simulink model "OpenLoop_simulation"  (R2022b)
settings: Solver=VariableStepAuto  StartTime=0.0  StopTime=5  RelTol=1e-3
values from neighbouring files (symbols this model uses):
  b = 0    [step_response_nominal.m]
  L = 0.23e-3    (= 0.00023)    [step_response_nominal.m]
  R = 3.85    [step_response_nominal.m]
  Stepsize = 0.5    [step_response_nominal.m]    (also in step_response_our.m)
  Tcomp = 0.0005*Ts*14    (= 7e-06)    [step_response_nominal.m]    (also in step_response_our.m)
  Ts = 0.001    [step_response_nominal.m]    (also in step_response_our.m)
settings Model: Creator=Alex Zhen  LastModifiedBy=lenovo
settings SolverCC: ZeroCrossAlgorithm=Adaptive
settings DebuggingCC: IgnoredZcDiagnostic=none

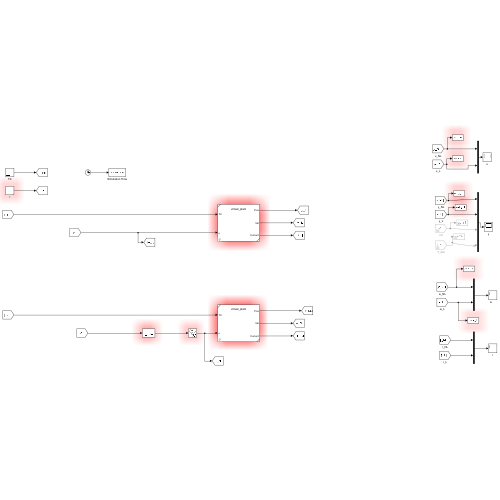
[thumbnail: Simulink's stored preview of the top-level diagram]
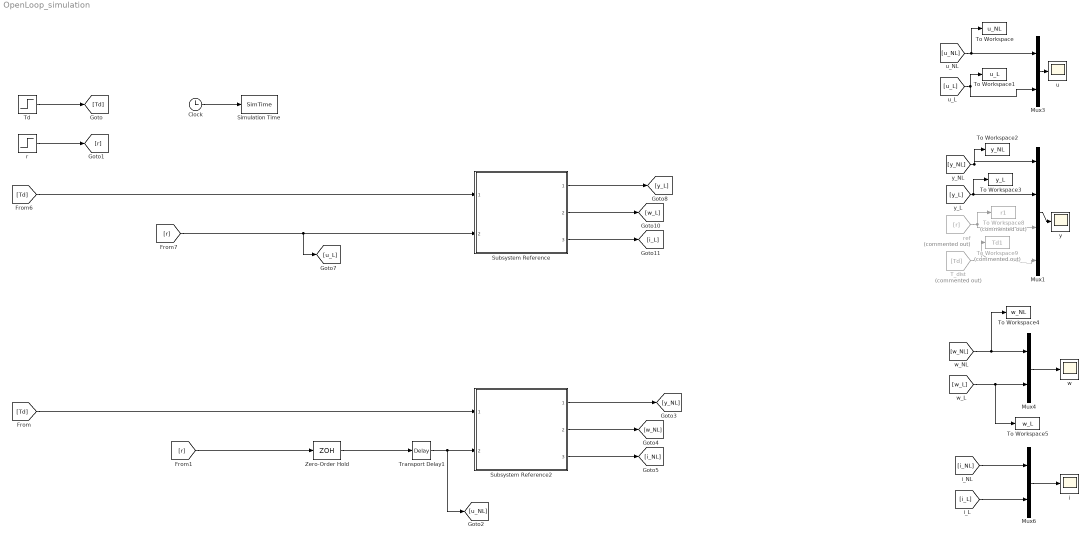
== system OpenLoop_simulation ==
  Clock : Clock
  Mux1 : Mux
  Mux3 : Mux  Inputs=2
  Mux4 : Mux  Inputs=2
  Mux6 : Mux  Inputs=2
  Simulation Time : ToWorkspace  VariableName=SimTime  SampleTime=-1
  Subsystem Reference : Subsystem  ReferencedSubsystem=virtual_plant  L=L  K_m=K_m  J_pend=J_pend  b=b  V_s=V_s  R=R  K_pend=K_pend  K_sin=K_sin  K_g=K_g  linear_mode=Linear
  Subsystem Reference2 : Subsystem  ReferencedSubsystem=virtual_plant  L=L  K_m=K_m  J_pend=J_pend  b=b  V_s=V_s  R=R  K_pend=K_pend  K_sin=K_sin  K_g=K_g  linear_mode=Linear
  T_dist : From  Commented=on  GotoTag=Td
  Td : Step  Time=5  After=0  SampleTime=0
  To Workspace : ToWorkspace  VariableName=u_NL  SampleTime=Ts
  To Workspace1 : ToWorkspace  VariableName=u_L  SampleTime=Ts
  To Workspace2 : ToWorkspace  VariableName=y_NL  SampleTime=Ts
  To Workspace3 : ToWorkspace  VariableName=y_L  SampleTime=Ts
  To Workspace4 : ToWorkspace  VariableName=w_NL  SampleTime=Ts
  To Workspace5 : ToWorkspace  VariableName=w_L  SampleTime=Ts
  To Workspace8 : ToWorkspace  Commented=on  VariableName=r1  SampleTime=Ts
  To Workspace9 : ToWorkspace  Commented=on  VariableName=Td1  SampleTime=Ts
  Transport Delay1 : TransportDelay  DelayTime=Tcomp  BufferSize=4096  PadeOrder=2
  Zero-Order Hold : ZeroOrderHold  SampleTime=Ts
  i : Scope
  r : Step  After=Stepsize  SampleTime=Ts
  ref : From  Commented=on  GotoTag=r
  u : Scope
  "w\t" : Scope
  y : Scope
  wires:
  Subsystem Reference2/1 -> [y_NL]
  Subsystem Reference/2 -> [w_L]
  Transport Delay1/1 -> [u_NL], Subsystem Reference2/2
  [Td] -> Subsystem Reference/1
  Zero-Order Hold/1 -> Transport Delay1/1
  Subsystem Reference/1 -> [y_L]
  Subsystem Reference/3 -> [i_L]
  Subsystem Reference2/3 -> [i_NL]
  [r] -> Zero-Order Hold/1
  r/1 -> [r]
  Td/1 -> [Td]
  [r] -> [u_L], Subsystem Reference/2
  Clock/1 -> Simulation Time/1
  Subsystem Reference2/2 -> [w_NL]
  [Td] -> Subsystem Reference2/1
  [i_NL] -> Mux6/1
  Mux6/1 -> i/1
  ref/1 -> To Workspace8/1, Mux1/3
  [i_L] -> Mux6/2
  Mux3/1 -> u/1
  Mux4/1 -> "w\t"/1
  [y_L] -> To Workspace3/1, Mux1/2
  [y_NL] -> To Workspace2/1, Mux1/1
  Mux1/1 -> y/1
  [u_L] -> To Workspace1/1, Mux3/2
  [u_NL] -> To Workspace/1, Mux3/1
  T_dist/1 -> To Workspace9/1, Mux1/4
  [w_NL] -> To Workspace4/1, Mux4/1
  [w_L] -> To Workspace5/1, Mux4/2
